simulink model "model_1"  (R2020b)
settings: Solver=ode45  StartTime=0.0  StopTime=120  RelTol=1e-3
model workspace (MAT data in the model file):
  b = 500
  m = 1000
  u = 150
settings Model: DataDictionary=MaiinPlantController_data.sldd  OrderedModelArguments=off  Creator=Diwakar Reddy  LastModifiedBy=Diwakar Reddy

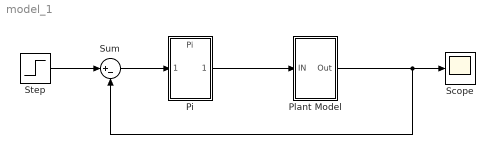
== system model_1 ==
  "Pi " : ModelReference  ModelNameDialog=Pi  SimulationMode=Normal  ModelReferenceVersion=1.5
  Plant Model : Subsystem
  Scope : Scope
  Step : Step  After=u  SampleTime=0
  Sum : Sum  Inputs=|+-
  wires:
  "Pi "/1 -> Plant Model/1(IN)
  Plant Model/1(Out) -> Scope/1, Sum/2
  Sum/1 -> "Pi "/1
  Step/1 -> Sum/1

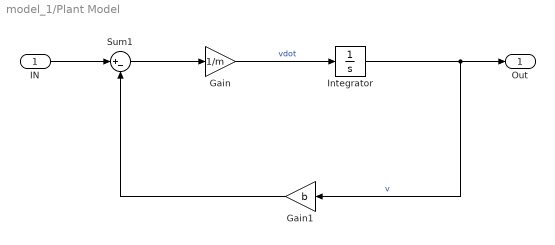
== system model_1/Plant Model ==
  IN : Inport
  Gain : Gain  Gain=1/m
  Gain1 : Gain  Gain=b
  Integrator : Integrator
  Sum1 : Sum  Inputs=|+-
  Out : Outport
  wires:
  Gain1/1 -> Sum1/2
  Integrator/1 -> Out/1, Gain1/1  "v"
  Sum1/1 -> Gain/1
  IN/1 -> Sum1/1
  Gain/1 -> Integrator/1  "vdot"
